simulink model "hcu_main_ADASwEPS"  (Simulink 8.2)
settings: Solver=FixedStepDiscrete  StartTime=0.0  StopTime=inf  FixedStep=0.001  RelTol=1e-3
PostLoadFcn:
  | , if any(exist('dsrtsu_mdlpostloadfcn', 'file') == [2, 3, 6]), try dsrtsu_mdlpostloadfcn('Execute', bdroot); catch fprintf('Error in PostLoadFcn (dsrtsu_mdlpostloadfcn) for model "%s":\n %s\n', bdroot, lasterr); end, end,
values from neighbouring files (symbols this model uses):
  C_TASK_1MS_S = (	C_TICK_TIME_S       )    [hcu_local_hdr.m]    (also in temp_ovrd_values.m = double(	0.001                  ))
  C_TICK_TIME_S = single(	0.005	    	)    [hcu_local_hdr.m]
  ENUM_EPSLFCSTATUS_ACTIVE = uint8(  2  )    [hcu_local_hdr.m]
  ENUM_EPSLFCSTATUS_TRANSITION = uint8(  3  )    [hcu_local_hdr.m]
  ENUM_EPSLKASTATUS_ACTIVE = uint8(  2  )    [hcu_local_hdr.m]
  ENUM_EPSMODEREQ_ANGLE = uint8(  1  )    [hcu_local_hdr.m]
  ENUM_EPSMODEREQ_INTERNAL = uint8(  0  )    [hcu_local_hdr.m]
  ENUM_EPSMODEREQ_TORQUE = uint8(  2  )    [hcu_local_hdr.m]
  ENUM_GEARPOSN_1ST = uint8(  1  )    [hcu_local_hdr.m]
  ENUM_GEARPOSN_2ND = uint8(  2  )    [hcu_local_hdr.m]
  ENUM_GEARPOSN_3RD = uint8(  3  )    [hcu_local_hdr.m]
  ENUM_GEARPOSN_4TH = uint8(  4  )    [hcu_local_hdr.m]
  ENUM_GEARPOSN_5TH = uint8(  5  )    [hcu_local_hdr.m]
  ENUM_GEARPOSN_6TH = uint8(  6  )    [hcu_local_hdr.m]
  ENUM_GEARPOSN_R = uint8(  7  )    [hcu_local_hdr.m]
  FALSE = boolean( 0 )    [hcu_local_hdr.m]
  TRUE = boolean( 1 )    [hcu_local_hdr.m]
undefined symbols (not defined in the file or in its folder): AISP_EPSCurrent_pct, AISP_TqASensorDelta_pct, AISP_TqBSensorDelta_pct, dHAL_IN, hal, INVALID_ABS1_TIMEOUT, INVALID_ABS2_TIMEOUT, INVALID_ABS3_TIMEOUT, INVALID_ABS4_TIMEOUT, INVALID_AC1_TIMEOUT, INVALID_ADASTORQ_REQ, INVALID_BCM1_TIMEOUT, INVALID_BCM2_TIMEOUT, INVALID_BOOSTER_VAC, INVALID_CSW1_TIMEOUT, INVALID_CUR_VEHDECE, INVALID_CURBRAKEDECE_REQ, INVALID_CURSTEERANG_REQ, INVALID_CURSTEERTQ_REQ, INVALID_ECM1_TIMEOUT, INVALID_ECM2_TIMEOUT, INVALID_ECM3_TIMEOUT, INVALID_ECM9_TIMEOUT, INVALID_ENG_TORQUE_FRICTIONAL, INVALID_ENG_TORQUE_INDICATED, INVALID_ENG_TORQUE_INDICATEDCOR, INVALID_ENG_TQ_MAX, INVALID_ENG_TQ_MIN, INVALID_EPAS2_TIMEOUT, INVALID_EPAS3_TIMEOUT, INVALID_EPB1_TIMEOUT, INVALID_EPS_BATTVOLT, INVALID_ESC_BATTVOLT, INVALID_GRADE, INVALID_HCU3_TIMEOUT, INVALID_HCU4_TIMEOUT, INVALID_HMI1_TIMEOUT, INVALID_HMI2_TIMEOUT, INVALID_LAT_ACC, INVALID_LONG_ACC, INVALID_MC_PRESSURE, INVALID_METER1_TIMEOUT, INVALID_METER3_TIMEOUT, INVALID_METER_VEHSPD, INVALID_ODO_METER, INVALID_OUTSIDE_TEMP, INVALID_PARKBRAKEBIND_STAT, INVALID_PEDALTQ_REQ, INVALID_SAS1_TIMEOUT, INVALID_SAS_ANGLE, INVALID_SHIFTER_POSN, INVALID_TCM1_TIMEOUT, INVALID_TCM2_TIMEOUT, INVALID_VCU1_TIMEOUT, INVALID_VCU2_TIMEOUT, INVALID_VEH_CRASH, INVALID_VEH_SPD, INVALID_WHEEL_SPD, INVALID_YAW_RATE, KHAL_MssgIdObj1_num ... (+8)
libraries: simulink x147, hcu_lib x38, rti1401lib_dio_type3 x4, rtimmsu_dsrtlib x3, app x1, rtiethernetudplib x1, rti1401lib_adc_type4 x1, rti1401lib_dac_type3 x1, inp x1, lidr x1, outp x1
(part 4 of 15)

== system hcu_main_ADASwEPS/ISP ==
  Hw_In : Inport
  CAN_In : Inport  Port=2
  trig_ISP : TriggerPort  TriggerType=function-call
  AngleProcessing : Subsystem
  Bus Selector1 : BusSelector  OutputSignals=ABS2.VehSpeed,ADAS1.ADAS_StrAngReq_A,ADAS1.ADAS_StrAngReq,ADAS1.ADAS_LFCTranGain_A,ADAS1.ADAS_LFCTransGain,ABS4.LatAccel,ADAS1.ADAS_StrTqReq_A,ADAS1.ADAS_StrTqReq,ADAS1.ADAS_EPSMode,ADAS1.ADAS_LKAStatus,ADAS1.ADAS_LFCStatus
  Bus Selector2 : BusSelector  OutputSignals=VHAL_EPSCurrent_pct
  Bus Selector3 : BusSelector  OutputSignals=VHAL_TqSensorADuty_pct,VHAL_TqSensorBDuty_pct
  Bus Selector4 : BusSelector  OutputSignals=VHAL_RelStrAng_deg
  Bus Selector5 : BusSelector  OutputSignals=VHAL_RelStrAng_deg
  Bus Selector6 : BusSelector  OutputSignals=ABS2.VehSpeed,ABS4.YawRate,ABS4.YawRate_V,ABS3.LR_RawWhlSpeed,ABS3.LR_RawWhlSpeed_V,ABS3.RR_RawWhlSpeed,ABS3.RR_RawWhlSpeed_V
  Bus Selector7 : BusSelector  OutputSignals=VHAL_EPSMotorSpd_rpm,VHAL_RelStrAng_deg
  ISP_Bus : BusCreator  Inputs=20
  KISP_EPSZeroReset_flg : Constant  Value=0
  Logical Operator1 : Logic  Operator=NOT  AllPortsSameDT=off  OutDataTypeStr=boolean
  Logical Operator2 : Logic  Operator=NOT  AllPortsSameDT=off  OutDataTypeStr=boolean
  Logical Operator3 : Logic  Operator=NOT  AllPortsSameDT=off  OutDataTypeStr=boolean
  MISP_EPSCurrent_A : Lookup  InputValues=AISP_EPSCurrent_pct  Table=MISP_EPSCurrent_A  LookUpMeth=Interpolation-Use End Values
      settings: AttributesFormatString="Input=\"%<InputValues>\"\\nOutput=\"%<Table>\""
  PassThrough : Subsystem
  TqProcessing : Subsystem
  ISP_Out : Outport
  wires:
  MISP_EPSCurrent_A/1 -> ISP_Bus/1  "VISP_EPSCurrent_A"
  KISP_EPSZeroReset_flg/1 -> AngleProcessing/1(KISP_EPSZeroReset_flg), TqProcessing/3(KISP_EPSZeroReset_flg)
  Hw_In/1 -> Bus Selector3/1, Bus Selector4/1, [Hw_In], Bus Selector2/1
  ISP_Bus/1 -> ISP_Out/1
  CAN_In/1 -> [CAN_In], Bus Selector1/1
  TqProcessing/1(VISP_EPSTqOnShaft_Nm) -> ISP_Bus/2
  TqProcessing/2(VISP_EPSTqOnShaftValid_flg) -> ISP_Bus/3
  AngleProcessing/1(VISP_StrAng_deg) -> ISP_Bus/4
  AngleProcessing/2(VISP_StrAngValid_flg) -> ISP_Bus/5
  Bus Selector1/1 -> PassThrough/2(VHAL_VehSpd_kph)  "<VehSpeed>"
  Logical Operator2/1 -> AngleProcessing/5(VHAL_YawRateValid_flg)
  Logical Operator3/1 -> AngleProcessing/9(VHAL_RRRawWhlSpdValid_flg)
  Logical Operator1/1 -> AngleProcessing/7(VHAL_LRRawWhlSpdValid_flg)
  PassThrough/1(VISP_StrAngSensorValid_flg) -> ISP_Bus/6
  Bus Selector1/3 -> PassThrough/4(VHAL_StrAngReq_deg)  "<ADAS_StrAngReq>"
  Bus Selector1/2 -> PassThrough/3(VHAL_StrAngReqAppl_flg)  "<ADAS_StrAngReq_A>"
  PassThrough/3(VISP_StrAngReq_deg) -> ISP_Bus/8
  PassThrough/2(VISP_StrAngReqAppl_flg) -> ISP_Bus/7
  PassThrough/4(VISP_VehSpd_kph) -> ISP_Bus/9
  PassThrough/5(VISP_RelStrAng_deg) -> ISP_Bus/10
  Bus Selector1/5 -> PassThrough/6(VHAL_LFCTransGain_rat)  "<ADAS_LFCTransGain>"
  Bus Selector1/4 -> PassThrough/5(VHAL_LFCTransGainAppl_flg)  "<ADAS_LFCTranGain_A>"
  PassThrough/7(VISP_LFCTransGain_rat) -> ISP_Bus/12
  PassThrough/6(VISP_LFCTransGainAppl_flg) -> ISP_Bus/11
  Bus Selector1/6 -> PassThrough/7(VHAL_LatAccel_mps2)  "<LatAccel>"
  PassThrough/8(VISP_LatAccel_mps2) -> ISP_Bus/13
  Bus Selector1/7 -> PassThrough/8(VHAL_StrTqReqAppl_flg)  "<ADAS_StrTqReq_A>"
  Bus Selector1/8 -> PassThrough/9(VHAL_StrTqReq_Nm)  "<ADAS_StrTqReq>"
  PassThrough/9(VISP_StrTqReqAppl_flg) -> ISP_Bus/14
  PassThrough/10(VISP_StrTqReq_Nm) -> ISP_Bus/15
  PassThrough/14(VISP_EPSMotorSpd_rpm) -> ISP_Bus/19
  PassThrough/15(VISP_EPSMotorAng_deg) -> ISP_Bus/20
  Bus Selector2/1 -> MISP_EPSCurrent_A/1  "<VHAL_EPSCurrent_pct>"
  Bus Selector3/1 -> TqProcessing/1(VHAL_TqSensorADuty_pct)  "<VHAL_TqSensorADuty_pct>"
  Bus Selector3/2 -> TqProcessing/2(VHAL_TqSensorBDuty_pct)  "<VHAL_TqSensorBDuty_pct>"
  Bus Selector4/1 -> AngleProcessing/2(VHAL_RelStrAng_deg)  "<VHAL_RelStrAng_deg>"
  Bus Selector5/1 -> PassThrough/1(VHAL_RelStrAng_deg)  "<VHAL_RelStrAng_deg>"
  [Hw_In] -> Bus Selector5/1
  [CAN_In] -> Bus Selector6/1
  Bus Selector6/1 -> AngleProcessing/3(VHAL_VehSpd_kph)  "<VehSpeed>"
  Bus Selector6/2 -> AngleProcessing/4(VHAL_YawRate_degps)  "<YawRate>"
  Bus Selector6/3 -> Logical Operator2/1  "<YawRate_V>"
  Bus Selector6/4 -> AngleProcessing/6(VHAL_LRRawWhlSpd_kph)  "<LR_RawWhlSpeed>"
  Bus Selector6/5 -> Logical Operator1/1  "<LR_RawWhlSpeed_V>"
  Bus Selector6/6 -> AngleProcessing/8(VHAL_RRRawWhlSpd_kph)  "<RR_RawWhlSpeed>"
  Bus Selector6/7 -> Logical Operator3/1  "<RR_RawWhlSpeed_V>"
  [Hw_In] -> Bus Selector7/1
  Bus Selector7/1 -> PassThrough/13(VHAL_EPSMotorSpd_rpm)  "<VHAL_EPSMotorSpd_rpm>"
  Bus Selector7/2 -> PassThrough/14(VHAL_EPSMotorAng_deg)  "<VHAL_RelStrAng_deg>"
  Bus Selector1/9 -> PassThrough/10(VHAL_EPSModeReq_enum)  "<ADAS_EPSMode>"
  Bus Selector1/10 -> PassThrough/11(VHAL_ADASLKAStatus_enum)  "<ADAS_LKAStatus>"
  Bus Selector1/11 -> PassThrough/12(VHAL_ADASLFCStatus_enum)  "<ADAS_LFCStatus>"
  PassThrough/11(VISP_EPSModeReq_enum) -> ISP_Bus/16
  PassThrough/12(VISP_ADASLKAStatus_enum) -> ISP_Bus/17
  PassThrough/13(VISP_ADASLFCStatus_enum) -> ISP_Bus/18

== system hcu_main_ADASwEPS/OSP ==
  BISP_outputs : Inport
  BEPSS_outputs : Inport  Port=2
  trig_OSP : TriggerPort  TriggerType=function-call
  Abs : Abs
  Bus Creator : BusCreator  Inputs=2
  Bus Selector : BusSelector  OutputSignals=VOSP_MotorDuty_pct
  Compare To Zero : simulink/Logic and Bit Operations/Compare To Zero  relop=>=  OutDataTypeStr=boolean
  Constant : Constant  Value=C_TASK_1MS_S
  Down_Rate : Constant  Value=-5
  Gain3 : Gain  Gain=1/100*4.5
  IsInRange : hcu_lib/IsInRange  SystemSampleTime=-1
  Negative : Constant  OutDataTypeStr=boolean
  Negative_Duty_Thres : Constant  Value=-5
  OSP : Subsystem
  Positive : Constant  Value=0  OutDataTypeStr=boolean
  Positive_Duty_Thres : Constant  Value=5
  RateLimit : hcu_lib/RateLimit  SystemSampleTime=-1
  Saturation : Saturate  UpperLimit=4.5  LowerLimit=0
  Switch : Switch  Criteria=u2 ~= 0
  Switch1 : Switch  Criteria=u2 ~= 0
  Terminator : Terminator
  Up_Rate : Constant  Value=5
  OSP_Out : Outport
  BOSP_outputs : Outport  Port=2
  wires:
  Positive/1 -> Switch/1
  Negative/1 -> Switch/3
  Abs/1 -> Gain3/1
  Bus Creator/1 -> OSP_Out/1  "OSP_Out"
  BEPSS_outputs/1 -> OSP/2(BEPSS_outputs)
  Bus Selector/1 -> Abs/1, Compare To Zero/1, Switch1/3, IsInRange/1, RateLimit/1  "<VOSP_MotorDuty_pct>"
  OSP/1(BOSP_outputs) -> BOSP_outputs/1, Bus Selector/1
  BISP_outputs/1 -> OSP/1(BISP_outputs)
  Switch/1 -> Bus Creator/2  "EPSDirection_flg"
  Gain3/1 -> Saturation/1
  Positive_Duty_Thres/1 -> IsInRange/2
  Negative_Duty_Thres/1 -> IsInRange/3
  Constant/1 -> RateLimit/2
  IsInRange/1 -> Switch1/2
  RateLimit/1 -> Switch1/1
  Up_Rate/1 -> RateLimit/3
  Down_Rate/1 -> RateLimit/4
  Switch1/1 -> Terminator/1
  Compare To Zero/1 -> Switch/2
  Saturation/1 -> Bus Creator/1  "DAC_V"

== system hcu_main_ADASwEPS/RTI Data ==
  RTI Data Store : Subsystem  Tag="struct('private',struct('version',struct('dsVer',uint32(2),'dsVerCreation',uint32(2),'RTI',struct('ver','7.4','type','RTI1401')),'access',struct('type','Model','isPerm',1,'created',['17-Nov-2015 11:37:15'],'modified',['24-May-2016 14:27:39'],'location','')),'public',struct('main',struct('data',[]),'sub',struct('name',{{'hcu_main_ADASwEPS'}},'data',{{struct('TH',struct('thTaskInfo',struct('taskType',{'TIMER','HWINT','TMRINT','SWINT','GLINT'},'tasksNumOf',{1,1,0,0,0},'srcIds',{{'TIMERA'},{'BB_BYP_ETHT1M0I0S0'},{},{},{}},'taskNames',{{['Timer Task 1']},{['rti_ethernet_interface_name Interrupt [RX/TX]']},{},{},{}})),'th_tc',struct('dataType',{'TASK','TASK'},'taskGroupId',{'',''},'taskGroupList',{{},{}},'taskSchedulingPolicy',{'FCFS','FCFS'},'taskType',{'TIMER','HWINT'},'blkh',{-1,['hcu_main_ADASwEPS/ETHERNET_UDP_SETUP_BL1/Common Hardware' char(10) 'Interrupt Interface']},'srcId',{'TIMERA','BB_BYP_ETHT1M0I0S0'},'srcSgnName',{['Timer A interrupt'],['BB_BYP_ETH Type 1 Module 1 HW-Int 0 Interrupt 0']},'srcCpuName',{'',''},'taskName',{['Timer Task 1  [0.001] s'],['rti_ethernet_interface_name Interrupt [RX/TX]']},'taskNameDisplayExt',{'',''},'smplTime',{0.001,0},'smplTimeOffs',{0,0},'hasFixedPriority',{0,0},'priority',{1,2},'hasFixedOvc',{0,0},'ovcType',{1,1},'ovcMax',{1,1}),'tc_th',struct('dataType',{'TASK','TASK'},'taskGroupId',{'',''},'taskGroupList',{{},{}},'taskSchedulingPolicy',{'FCFS','FCFS'},'taskType',{'TIMER','HWINT'},'blkh',{-1,['hcu_main_ADASwEPS/ETHERNET_UDP_SETUP_BL1/Common Hardware' char(10) 'Interrupt Interface']},'srcId',{'TIMERA','BB_BYP_ETHT1M0I0S0'},'srcSgnName',{['Timer A interrupt'],['BB_BYP_ETH Type 1 Module 1 HW-Int 0 Interrupt 0']},'srcCpuName',{'',''},'taskName',{['Timer Task 1  [0.001] s'],['rti_ethernet_interface_name Interrupt [RX/TX]']},'taskNameDisplayExt',{'',''},'smplTime',{0.001,0},'smplTimeOffs',{0,0},'hasFixedPriority',{0,0},'priority',{1,2},'hasFixedOvc',{0,0},'ovcType',{1,1},'ovcMax',{1,1}))}})))"  mask(RTI_DATA_STORE){}
      mask help:
      | RTI Data Store Block. This block is used by RTI to store internal model dependent data. Deleting this block will result in data loss.
      |
      | NEVER DELETE, COPY, OR MODIFY THIS BLOCK!
      mask Help:
      | RTI Data Store Block. This block is used by RTI to store internal model dependent data. Deleting this block will result in data loss.
      | 
      | NEVER DELETE, COPY, OR MODIFY THIS BLOCK!
      mask Display: text(0.5, 0.5, ' ', 'HorizontalAlignment', 'center');

== system hcu_main_ADASwEPS/RTICANMM ControllerSetup ==
  VariationInput : Inport
  Reset : Inport  Port=2
  ModelClose : Subsystem  mask(RTICANMMModelClose){}
  RTICANMMCHANNEL_TLC : S-Function  FunctionName=rticanmm_tlc_adv  Parameters=1401,1,1,0,500,'unused'  EnableBusSupport=off  mask(RTICANMMCHANNEL_TLC){}
  Variation_DTC : DataTypeConversion  SaturateOnIntegerOverflow=on  RndMeth=Zero
  sfcn : S-Function  InitFcn=rticanmm_initfcn(gcb, 'SFCNs')  FunctionName=RTICANMM_SETUP_CAN_1  EnableBusSupport=off
      mask init:
      | rticanmm_initfcn(gcb, 'SFCNs')
  wires:
  Reset/1 -> sfcn/2
  VariationInput/1 -> Variation_DTC/1
  Variation_DTC/1 -> sfcn/1

== system hcu_main_ADASwEPS/RTICANMM ControllerSetup1 ==
  VariationInput : Inport
  Reset : Inport  Port=2
  ModelClose : Subsystem  mask(RTICANMMModelClose){}
  RTICANMMCHANNEL_TLC : S-Function  FunctionName=rticanmm_tlc_adv  Parameters=1401,1,2,0,500,'unused'  EnableBusSupport=off  mask(RTICANMMCHANNEL_TLC){}
  Variation_DTC : DataTypeConversion  SaturateOnIntegerOverflow=on  RndMeth=Zero
  sfcn : S-Function  InitFcn=rticanmm_initfcn(gcb, 'SFCNs')  FunctionName=RTICANMM_SETUP_CAN_2  EnableBusSupport=off
      mask init:
      | rticanmm_initfcn(gcb, 'SFCNs')
  wires:
  Reset/1 -> sfcn/2
  VariationInput/1 -> Variation_DTC/1
  Variation_DTC/1 -> sfcn/1

== system hcu_main_ADASwEPS/RTICANMM GeneralSetup ==
  ModelClose : Subsystem  mask(RTICANMMModelClose){}
  TRC Exclusion : rtimmsu_dsrtlib/TRC Exclusion

== system hcu_main_ADASwEPS/Triggering2CAN1 ==
  ADAS4 : Subsystem
  ADAS5 : Subsystem
  buscreator : BusCreator  Inputs=2
  out : Outport
  wires:
  ADAS4/1(out) -> buscreator/1  "ADAS4"
  ADAS5/1(out) -> buscreator/2  "ADAS5"
  buscreator/1 -> out/1  "CAN"

== system hcu_main_ADASwEPS/User2CAN1_ ==
  BOSP_outputs : Inport
  BOUTP_outputs : Inport  Port=2  OutDataTypeStr=Bus: BOUTP_outputs
  ADAS1 : Subsystem
  ADAS2 : Subsystem
  ADAS3 : Subsystem
  ADAS4 : Subsystem
  ADAS5 : Subsystem
  EPAS2 : Subsystem
  EPAS3 : Subsystem
  SAS1 : Subsystem
  buscreator : BusCreator  Inputs=8
  out : Outport
  wires:
  ADAS1/1(out) -> buscreator/1  "ADAS1"
  ADAS2/1(out) -> buscreator/2  "ADAS2"
  ADAS3/1(out) -> buscreator/3  "ADAS3"
  ADAS4/1(out) -> buscreator/4  "ADAS4"
  ADAS5/1(out) -> buscreator/5  "ADAS5"
  EPAS2/1(out) -> buscreator/6  "EPAS2"
  EPAS3/1(out) -> buscreator/7  "EPAS3"
  SAS1/1(out) -> buscreator/8  "SAS1"
  buscreator/1 -> out/1  "CAN"
  BOSP_outputs/1 -> EPAS2/1(BOSP_outputs), SAS1/1(BOSP_outputs), EPAS3/1(BOSP_outputs)
  BOUTP_outputs/1 -> ADAS1/1(BOUTP_outputs), ADAS2/1(BOUTP_outputs), ADAS3/1(BOUTP_outputs), ADAS5/1(BOUTP_outputs), ADAS4/1(BOUTP_outputs)

== system hcu_main_ADASwEPS/User2CAN2 ==
  CAN1_Rx : Inport
  ABS2_C : Subsystem
  ABS4_C : Subsystem
  BCM1_C : Subsystem
  CSW1_C : Subsystem
  FECU1_C : Subsystem
  SAS1_C : Subsystem
  SpeedInformation : Subsystem
  YawRateInformation : Subsystem
  buscreator : BusCreator  Inputs=8
  out : Outport
  wires:
  ABS2_C/1(out) -> buscreator/1  "ABS2_C"
  ABS4_C/1(out) -> buscreator/2  "ABS4_C"
  BCM1_C/1(out) -> buscreator/3  "BCM1_C"
  CSW1_C/1(out) -> buscreator/4  "CSW1_C"
  FECU1_C/1(out) -> buscreator/5  "FECU1_C"
  SAS1_C/1(out) -> buscreator/6  "SAS1_C"
  SpeedInformation/1(out) -> buscreator/7  "SpeedInformation"
  YawRateInformation/1(out) -> buscreator/8  "YawRateInformation"
  buscreator/1 -> out/1  "CAN"
  CAN1_Rx/1 -> YawRateInformation/1(CAN1_Rx), SpeedInformation/1(CAN1_Rx), SAS1_C/1(CAN1_Rx), FECU1_C/1(CAN1_Rx), CSW1_C/1(CAN1_Rx), BCM1_C/1(CAN1_Rx), ABS4_C/1(CAN1_Rx), ABS2_C/1(CAN1_Rx1)
